simulink model "Bonus"  (R2020a)
settings: Solver=FixedStepAuto  StartTime=0.0  StopTime=10.0  FixedStep=1e-3  RelTol=1e-3  EnableMultiTasking=on
model workspace (MAT data in the model file):
  PWM_duty_cycle = 5
libraries: frdmk64flib x2
settings Model: ExtModeTrigDuration=5  Creator=theodor  LastModifiedBy=theodor
settings OptimizationCC: EnhancedBackFolding=on  PassReuseOutputArgsAs=Individual arguments  ZeroExternalMemoryAtStartup=off  ZeroInternalMemoryAtStartup=off  MaxStackSize=64  OptimizeBlockOrder=speed  DifferentSizesBufferReuse=on  OptimizationCustomize=off  EfficientTunableParamExpr=on
settings DebuggingCC: ParameterTunabilityLossMsg=error
settings HardwareCC: ProdBitPerPointer=32  ProdBitPerSizeT=32  ProdBitPerPtrDiffT=32  ProdLargestAtomicInteger=Long  ProdLargestAtomicFloat=Double  ProdWordSize=32  ProdHWDeviceType=ARM Compatible->ARM Cortex
settings SFSimCC: MATLABDynamicMemAlloc=off
settings RTWCC: SystemTargetFile=ert.tlc  HardwareBoard=NXP FRDM-K64F  TemplateMakefile=ert_default_tmf  Toolchain=GNU Tools for ARM Embedded Processors
settings CodeAppCC: ForceParamTrailComments=on  IgnoreCustomStorageClasses=off  OperatorAnnotations=on  SimulinkDataObjDesc=on  SFDataObjDesc=on  InsertBlockDesc=on

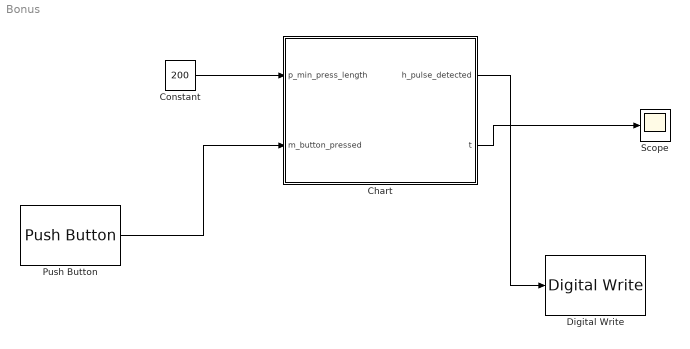
== system Bonus ==
  Chart : Stateflow chart  TreatAsAtomicUnit=on
  Constant : Constant  Value=200
  Digital Write : frdmk64flib/Digital Write  Whichpin=RED_LED
  Push Button : frdmk64flib/Push Button  Whichswitch=SW3  SampleTime1=-1
  Scope : Scope
  wires:
  Push Button/1 -> Chart/2(m_button_pressed)
  Constant/1 -> Chart/1(p_min_press_length)
  Chart/1(h_pulse_detected) -> Digital Write/1
  Chart/2(t) -> Scope/1

== stateflow chart Bonus/Chart ==
  state INVALID_PULSE
  state IDLE
    entry:
    h_pulse_detected = 0;
  state BUTTON_DOWN
    exit:
    t = elapsed(msec);
  state VALID_PULSE
    entry:
    h_pulse_detected = 1;
    t = t + elapsed(msec)
  INVALID_PULSE -> IDLE : [~m_button_pressed]
  BUTTON_DOWN -> INVALID_PULSE [order 2] : after(p_min_press_length,msec)
  (default) -> IDLE
  IDLE -> BUTTON_DOWN : [m_button_pressed]
  VALID_PULSE -> IDLE : after(10,msec)
  BUTTON_DOWN -> VALID_PULSE [order 1] : [~m_button_pressed]
  data: p_min_press_length input; h_pulse_detected output int8; m_button_pressed input boolean; t output
